simulink model "TestLQR3"  (R2017a)
settings: Solver=ode3  StartTime=0.0  StopTime=20  FixedStep=4e-3  MaxStep=1e-2  RelTol=1e-3
values from neighbouring files (symbols this model uses):
  A = transpose(A)    [modelM1.m]
  B = transpose(c)    [modelM1.m]
  C = transpose(b)    [modelM1.m]
libraries: simulink x2
settings Model: Creator=Rosa Garrido  LastModifiedBy=David
settings DataIOCC: SaveFormat=StructureWithTime
settings OptimizationCC: LifeSpan=inf
settings DebuggingCC: SFExecutionAtInitializationDiag=none
settings HardwareCC: ProdBitPerSizeT=32  ProdBitPerPtrDiffT=32  ProdWordSize=32  ProdHWDeviceType=Specified

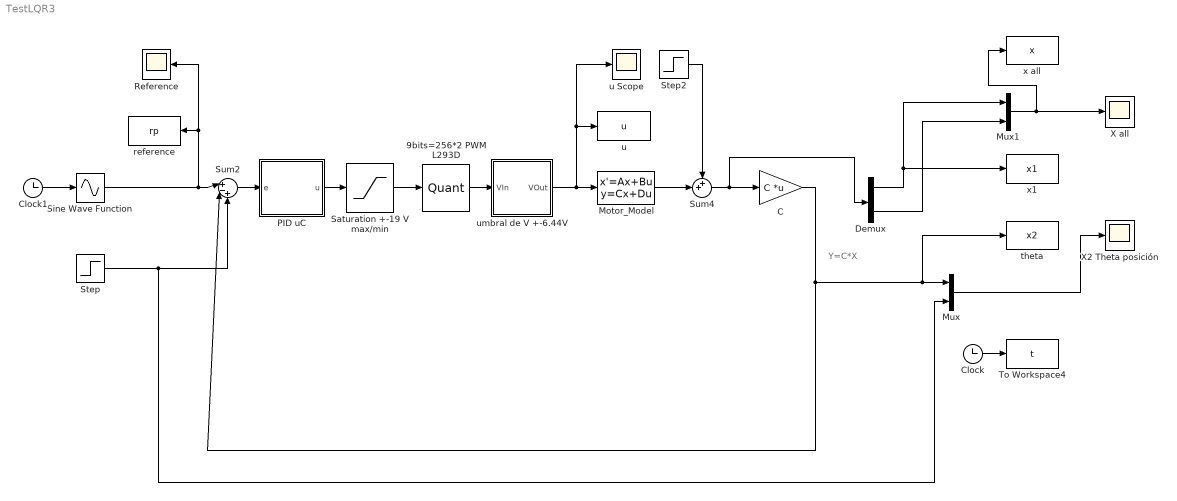
== system TestLQR3 ==
  note: Y=C*X
  9bits=256*2 PWM L293D : Quantizer  QuantizationInterval=0.0781
  C : Gain  Gain=C  Multiplication=Matrix(K*u)
  Clock : Clock
  Clock1 : Clock
  Demux : Demux  Outputs=2
  Motor_Model : StateSpace  A=A  B=B  C=eye(2)  D=zeros(2,1)  X0=[0 -1.6926*3*0]
  Mux : Mux  Inputs=2
  Mux1 : Mux  Inputs=2
  PID uC : Subsystem
  Reference : Scope
  Saturation +-19 V max/min : Saturate  UpperLimit=19  LowerLimit=-19
  Sine Wave Function : Sin  TimeSource=Use external signal  Amplitude=0  SampleTime=0
  Step : Step  Time=0  After=45  SampleTime=0
  Step2 : Step  Time=10  After=0.2  SampleTime=0
  Sum2 : Sum  Inputs=|+-+
  Sum4 : Sum  Inputs=++|
  To Workspace4 : ToWorkspace  VariableName=t  SampleTime=-1
      settings: Save2DSignal=2-D array (concatenate along first dimension)
  X all : Scope
  X2 Theta posición : Scope
  reference : ToWorkspace  VariableName=rp  SampleTime=-1
      settings: Save2DSignal=2-D array (concatenate along first dimension)
  theta : ToWorkspace  VariableName=x2  SampleTime=-1
      settings: Save2DSignal=2-D array (concatenate along first dimension)
  u : ToWorkspace  VariableName=u  SampleTime=-1
      settings: Save2DSignal=2-D array (concatenate along first dimension)
  u Scope : Scope
  umbral de V +-6.44V : Subsystem
  x all : ToWorkspace  VariableName=x  SampleTime=-1
      settings: Save2DSignal=2-D array (concatenate along first dimension)
  x1 : ToWorkspace  VariableName=x1  SampleTime=-1
      settings: Save2DSignal=2-D array (concatenate along first dimension)
  wires:
  Clock/1 -> To Workspace4/1
  Mux1/1 -> x all/1, X all/1
  Demux/1 -> x1/1, Mux1/1
  Demux/2 -> Mux1/2
  Motor_Model/1 -> Sum4/2
  Step2/1 -> Sum4/1
  Sum4/1 -> Demux/1, C/1
  umbral de V +-6.44V/1(VOut) -> u/1, u Scope/1, Motor_Model/1
  C/1 -> theta/1, Mux/1, Sum2/2
  Clock1/1 -> Sine Wave Function/1
  Mux/1 -> X2 Theta posición/1
  Sine Wave Function/1 -> reference/1, Reference/1, Sum2/1
  Step/1 -> Mux/2, Sum2/3
  9bits=256*2 PWM L293D/1 -> umbral de V +-6.44V/1(VIn)
  Saturation +-19 V max/min/1 -> 9bits=256*2 PWM L293D/1
  Sum2/1 -> PID uC/1(e)
  PID uC/1(u) -> Saturation +-19 V max/min/1

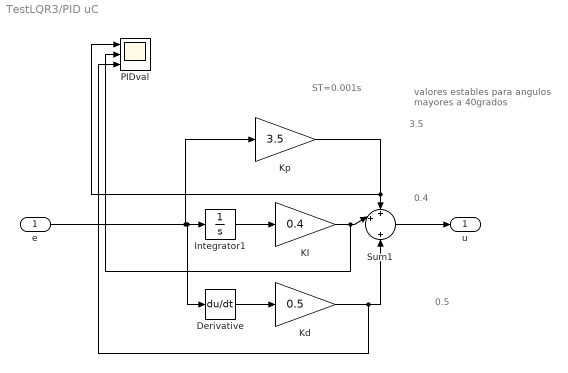
== system TestLQR3/PID uC ==
  note: ST=0.001s
  note: valores estables para angulos
      | mayores a 40grados
  note: 0.5
  note: 0.4
  note: 3.5
  e : Inport
  Derivative : Derivative
  Integrator1 : Integrator
  KI : Gain  Gain=0.4
  Kd : Gain  Gain=0.5
  Kp : Gain  Gain=3.5
  PIDval : Scope  NumInputPorts=3
  Sum1 : Sum  Inputs=++|+
  u : Outport
  wires:
  e/1 -> Integrator1/1, Derivative/1, Kp/1
  Integrator1/1 -> KI/1
  Kp/1 -> PIDval/1, Sum1/1
  KI/1 -> PIDval/2, Sum1/2
  Derivative/1 -> Kd/1
  Sum1/1 -> u/1
  Kd/1 -> PIDval/3, Sum1/3

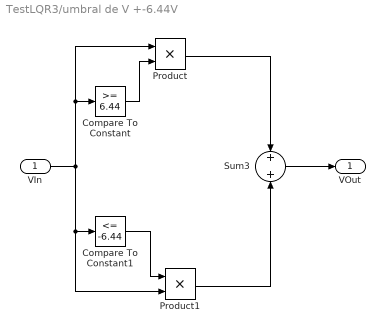
== system TestLQR3/umbral de V +-6.44V ==
  VIn : Inport
  Compare To Constant : simulink/Logic and Bit Operations/Compare To Constant  relop=>=  const=6.44  OutDataTypeStr=boolean
  Compare To Constant1 : simulink/Logic and Bit Operations/Compare To Constant  relop=<=  const=-6.44  OutDataTypeStr=boolean
  Product : Product
  Product1 : Product
  Sum3 : Sum  Inputs=+|+
  VOut : Outport
  wires:
  Compare To Constant1/1 -> Product1/1
  VIn/1 -> Product/1, Compare To Constant/1, Product1/2, Compare To Constant1/1
  Product/1 -> Sum3/1
  Product1/1 -> Sum3/2
  Compare To Constant/1 -> Product/2
  Sum3/1 -> VOut/1
